simulink library "commsrccod"  (Simulink 5.0)
libraries: commsrccod x2
settings Model: Creator=mikem  LastModifiedBy=mmclerno

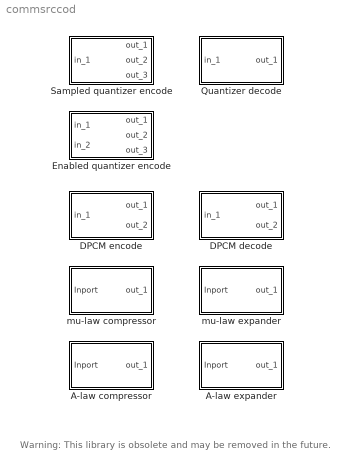
== system commsrccod ==
  note: Warning:  This library is obsolete and may be
      | removed in the future.
  A-law compressor : Subsystem  mask(A-law compressor){A=87.6, V=1}
      mask prompts: A "A value:"; V "Peak signal magnitude:"
      mask help: Compress the input signal using A-law compressor. The A-law compressor uses logarithm computation.
      mask init:
      | lnA1=log(A)+1;AdlnA1=A/lnA1;VdlnA1=V/lnA1;VdA=V/A;AdV=A/V;
      mask Help: This block processes a vector signal. The output has the same length as the input signal. The prevailing value for A is A=87.6.
      mask Display: disp('A-law\ncompressor')
  A-law expander : Subsystem  mask(A-law expander){A=87.6, V=1}
      mask prompts: A "A value:"; V "Signal peak magnitude:"
      mask help: Inverse computation of A-law compressor.
      mask init:
      | lnA1=log(A)+1;VdlnA1=V/lnA1;lnA1dA=lnA1/A;lnA1dV=lnA1/V;VdA=V/A;
      mask Help: This block reverses the computation with A-law compressor. The prevailing value for A is A=87.6.
      mask Display: disp('A-law\nexpander')
  DPCM decode : Subsystem  mask(DPCM decode){num=[0 .9963], den=1, codebook=[-.0848 -.029 .0298 .0853], sample_time=.1}
      mask prompts: num "Predictor transfer function numerator:"; den "Predictor transfer function denominator:"; codebook "Quantization codebook:"; sample_time "Sample time (sec):"
      mask help: Input the DPCM coded index. Output DPCM decodes to the 1st outport and quantization decode to the 2nd outport.
      mask Help: This block recovers the source code using the DPCM decode method. The parameters in this block should match the parameters in the DPCM encoder.
      mask Display: disp('DPCM\ndecode')
  DPCM encode : Subsystem  mask(DPCM encode){num=[0 .9963], den=1, partition=[-.0569 .0004 .0576], codebook=[-.0848 -.029 .0298 .0853], sample_time=.1}
      mask prompts: num "Predictor numerator:"; den "Predictor denominator:"; partition "Quantization partition:"; codebook "Quantization codebook:"; sample_time "Sample time (sec):"
      mask help: Output the DPCM encoded index to the 1st outport and the quantization recovered value to the 2nd outport.
      mask Help: The 1st outport outputs the index of the predictive error. The 2nd outport outputs the predictive error. Use the DPCMOPT function for the FIR filter training. A delta modulation is a special case with the numerator as [0,x], the denominator as 1 for the\npredictor.
      mask Display: disp('DPCM\nencode')
  Enabled quantizer encode : Subsystem  mask(Scalar quantization encode){partition=[-.75 -.25 .25 .75], codebook=[-.825 -.5 0 .5 .825], n=2}
      mask prompts: partition "Quantization partition:"; codebook "Quantization codebook:"; n "Input signal vector length:"
      mask help: Triggered by 2nd input signal, this block quantize an analog signal to (1)digital signal, (2)quantization value, (3)distortion.
      mask init:
      | [x,y]=trigicon(0,25,get_param(gcb,'orientation'),1);
      mask Help: This block quantizes the first inport signal into quantization index (1st outport), quantized value (2nd outport), and distortion (3rd outport). This block uses scalar quantization method. The input signal to the 1st inport can be a vector. The operation of this block is enabled by the non-zero signal from the second inport. When the block is not enabled, the block keeps the last output value.
      mask Display: plot(0,0,100,100,x,y);disp('Quantizer')
  Quantizer decode : Subsystem  mask(Scalar quantization decode){codebook=[-.825 -.5 0, .5 .825]}
      mask prompts: codebook "Quantization codebook:"
      mask help: Output the value in the given codebook based on the input index value.
      mask Help: This block takes the quantized index as input and outputs the quantization value. The output vector size is the same as the input vector size. Inputs 0, 1, ..., N-1 lead to CK(1), CK(2), .. CK(N) output.
      mask Display: disp('Quantizer\ndecode')
  Sampled quantizer encode : Subsystem  mask(Scalar quantization encode){partition=[-.75 -.25 .25 .75], codebook=[-.825 -.5 0 .5 .825], n=2, sample_time=.1}
      mask prompts: partition "Quantization partition:"; codebook "Quantization codebook:"; n "Input signal vector length:"; sample_time "Sample time (sec):"
      mask help: Quantize an analog signal to (1)digital signal, (2)quantization value, and (3)distortion at every sample time point.
      mask Help: This block converts the input analog signal to digital signal (1st outport) with the quantized value (2nd outport), and distortion (3rd outport) at every sample point. The input signa can be a vector. When the sample time is a two-elements vector, the second element is the offset value. The length of the partition is one less than the length of codebook. Use LLOYDS to optimize the partition and codebook.
      mask Display: disp('Scalar\nquantizer')
  mu-law compressor : Subsystem  mask(mu-law compressor){mu=255, V=1}
      mask prompts: mu "mu value:"; V "Peak signal magnitude:"
      mask help: Compress the input signal using mu-law compressor. The mu-law compressor uses logarithm computation.
      mask init:
      | mudV=mu/V;Vln1mu=V/log(1+mu);
      mask Help: This block processes a vector signal. The output has the same length as the input signal. The prevailing value is mu=255.
      mask Display: disp('mu-law\ncompressor')
  mu-law expander : Subsystem  mask(mu-law expander){mu=255, V=1}
      mask prompts: mu "mu value:"; V "Signal peak magnitude:"
      mask help: Inverse computation of mu-law compressor.
      mask init:
      | Vmu=V/mu;ln1mdV=log(1+mu)/V;
      mask Help: This block reverses the computation with mu-law compressor. The prevailing value for mu is mu=255.
      mask Display: disp('mu-law\nexpander')

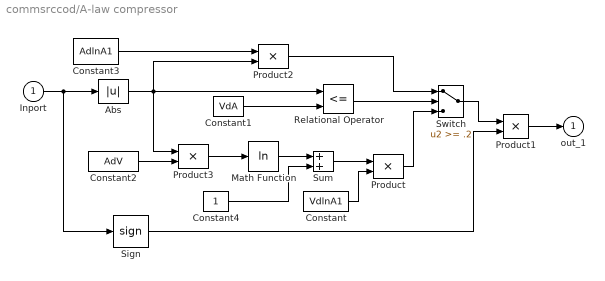
== system commsrccod/A-law compressor ==
  Inport : Inport
  Abs : Abs  SaturateOnIntegerOverflow=on
  Constant : Constant  Value=VdlnA1
  Constant1 : Constant  Value=VdA
  Constant2 : Constant  Value=AdV
  Constant3 : Constant  Value=AdlnA1
  Constant4 : Constant
  Math Function : Math  Operator=log
  Product{,1..3} (4 alike) : Product  SaturateOnIntegerOverflow=on  InputSameDT=on
  Relational Operator : RelationalOperator  Operator=<=  InputSameDT=on
  Sign : Signum
  Sum : Sum  SaturateOnIntegerOverflow=on  InputSameDT=on
  Switch : Switch  Threshold=.2  SaturateOnIntegerOverflow=on  InputSameDT=on
  out_1 : Outport  InitialOutput=0
  wires:
  Product1/1 -> out_1/1
  Inport/1 -> Sign/1, Abs/1
  Sign/1 -> Product1/2
  Switch/1 -> Product1/1
  Constant1/1 -> Relational Operator/2
  Relational Operator/1 -> Switch/2
  Product2/1 -> Switch/1
  Constant3/1 -> Product2/1
  Constant2/1 -> Product3/2
  Abs/1 -> Product3/1, Product2/2, Relational Operator/1
  Product3/1 -> Math Function/1
  Math Function/1 -> Sum/1
  Constant4/1 -> Sum/2
  Constant/1 -> Product/2
  Sum/1 -> Product/1
  Product/1 -> Switch/3

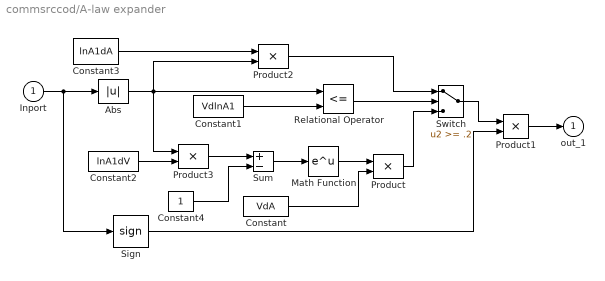
== system commsrccod/A-law expander ==
  Inport : Inport
  Abs : Abs  SaturateOnIntegerOverflow=on
  Constant : Constant  Value=VdA
  Constant1 : Constant  Value=VdlnA1
  Constant2 : Constant  Value=lnA1dV
  Constant3 : Constant  Value=lnA1dA
  Constant4 : Constant
  Math Function : Math
  Product{,1..3} (4 alike) : Product  SaturateOnIntegerOverflow=on  InputSameDT=on
  Relational Operator : RelationalOperator  Operator=<=  InputSameDT=on
  Sign : Signum
  Sum : Sum  Inputs=+-  SaturateOnIntegerOverflow=on  InputSameDT=on
  Switch : Switch  Threshold=.2  SaturateOnIntegerOverflow=on  InputSameDT=on
  out_1 : Outport  InitialOutput=0
  wires:
  Product/1 -> Switch/3
  Constant/1 -> Product/2
  Constant4/1 -> Sum/2
  Constant2/1 -> Product3/2
  Constant3/1 -> Product2/1
  Product2/1 -> Switch/1
  Abs/1 -> Product3/1, Product2/2, Relational Operator/1
  Relational Operator/1 -> Switch/2
  Constant1/1 -> Relational Operator/2
  Switch/1 -> Product1/1
  Sign/1 -> Product1/2
  Inport/1 -> Sign/1, Abs/1
  Product1/1 -> out_1/1
  Product3/1 -> Sum/1
  Sum/1 -> Math Function/1
  Math Function/1 -> Product/1

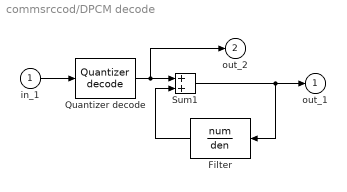
== system commsrccod/DPCM decode ==
  in_1 : Inport
  Filter : DiscreteFilter  Orientation=left  Numerator=num  Denominator=den  SampleTime=sample_time
  Quantizer decode : commsrccod/Quantizer decode  codebook=codebook
  Sum1 : Sum  SaturateOnIntegerOverflow=on  InputSameDT=on
  out_1 : Outport  InitialOutput=0
  out_2 : Outport  Port=2  InitialOutput=0
  wires:
  Quantizer decode/1 -> out_2/1, Sum1/1
  Sum1/1 -> Filter/1, out_1/1
  Filter/1 -> Sum1/2
  in_1/1 -> Quantizer decode/1

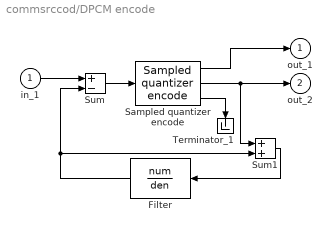
== system commsrccod/DPCM encode ==
  in_1 : Inport
  Filter : DiscreteFilter  Orientation=left  Numerator=num  Denominator=den  SampleTime=sample_time
  Sampled quantizer encode : commsrccod/Sampled quantizer encode  partition=partition  codebook=codebook  n=1  sample_time=sample_time
  Sum : Sum  Inputs=+-  SaturateOnIntegerOverflow=on  InputSameDT=on
  Sum1 : Sum  SaturateOnIntegerOverflow=on  InputSameDT=on
  Terminator_1 : Terminator
      settings: Orientation=down
  out_1 : Outport  InitialOutput=0
  out_2 : Outport  Port=2  InitialOutput=0
  wires:
  Sampled quantizer encode/3 -> Terminator_1/1
  Sampled quantizer encode/2 -> out_2/1, Sum1/1
  Sampled quantizer encode/1 -> out_1/1
  Sum/1 -> Sampled quantizer encode/1
  in_1/1 -> Sum/1
  Filter/1 -> Sum1/2, Sum/2
  Sum1/1 -> Filter/1

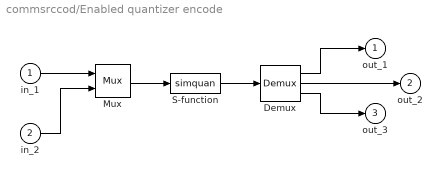
== system commsrccod/Enabled quantizer encode ==
  in_1 : Inport
  in_2 : Inport  Port=2
  Demux : Demux  Outputs=[n n n]
  Mux : Mux  Inputs=[n 1]
  S-function : S-Function  FunctionName=simquan  Parameters=n, partition, codebook
  out_1 : Outport  InitialOutput=0
  out_2 : Outport  Port=2  InitialOutput=0
  out_3 : Outport  Port=3  InitialOutput=0
  wires:
  Demux/3 -> out_3/1
  Demux/2 -> out_2/1
  Demux/1 -> out_1/1
  S-function/1 -> Demux/1
  Mux/1 -> S-function/1
  in_2/1 -> Mux/2
  in_1/1 -> Mux/1

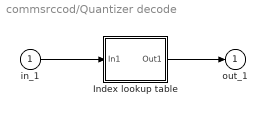
== system commsrccod/Quantizer decode ==
  in_1 : Inport
  Index lookup table : Subsystem  mask(No-intepret Lookup table){@1=codebook}
      mask prompts: @1 "Codebook:"
      mask help: Output one of the values in the look-up table.
      mask init:
      | codebook=@1;
      mask Help: When codebook is a matrix, the block input can only be a scalar. The block output the row with the column index provided in the input. When codebook is a vector, the block output the same length as the input vector. The output is one of the values in codebook with the index provided by the input.
      mask Display: disp('Index\nLookup tb')
  out_1 : Outport  InitialOutput=0
  wires:
  Index lookup table/1(Out1) -> out_1/1
  in_1/1 -> Index lookup table/1(In1)

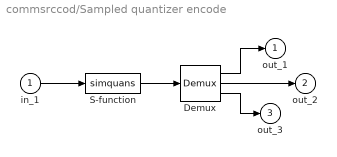
== system commsrccod/Sampled quantizer encode ==
  in_1 : Inport
  Demux : Demux  Outputs=[n n n]
  S-function : S-Function  FunctionName=simquans  Parameters=n, partition, codebook,sample_time
  out_1 : Outport  InitialOutput=0
  out_2 : Outport  Port=2  InitialOutput=0
  out_3 : Outport  Port=3  InitialOutput=0
  wires:
  in_1/1 -> S-function/1
  S-function/1 -> Demux/1
  Demux/1 -> out_1/1
  Demux/2 -> out_2/1
  Demux/3 -> out_3/1

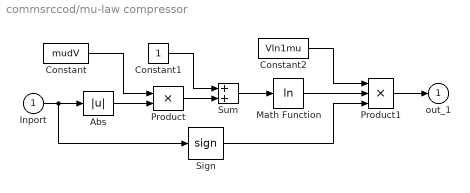
== system commsrccod/mu-law compressor ==
  Inport : Inport
  Abs : Abs  SaturateOnIntegerOverflow=on
  Constant : Constant  Value=mudV
  Constant1 : Constant
  Constant2 : Constant  Value=Vln1mu
  Math Function : Math  Operator=log
  Product : Product  SaturateOnIntegerOverflow=on  InputSameDT=on
  Product1 : Product  Inputs=3  SaturateOnIntegerOverflow=on  InputSameDT=on
  Sign : Signum
  Sum : Sum  SaturateOnIntegerOverflow=on  InputSameDT=on
  out_1 : Outport  InitialOutput=0
  wires:
  Product1/1 -> out_1/1
  Constant2/1 -> Product1/1
  Sign/1 -> Product1/3
  Math Function/1 -> Product1/2
  Inport/1 -> Sign/1, Abs/1
  Sum/1 -> Math Function/1
  Constant1/1 -> Sum/1
  Product/1 -> Sum/2
  Constant/1 -> Product/1
  Abs/1 -> Product/2

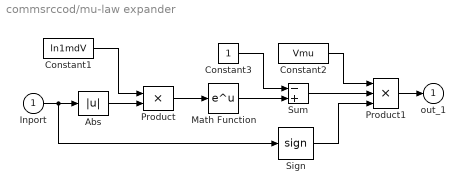
== system commsrccod/mu-law expander ==
  Inport : Inport
  Abs : Abs  SaturateOnIntegerOverflow=on
  Constant1 : Constant  Value=ln1mdV
  Constant2 : Constant  Value=Vmu
  Constant3 : Constant
  Math Function : Math
  Product : Product  SaturateOnIntegerOverflow=on  InputSameDT=on
  Product1 : Product  Inputs=3  SaturateOnIntegerOverflow=on  InputSameDT=on
  Sign : Signum
  Sum : Sum  Inputs=-+  SaturateOnIntegerOverflow=on  InputSameDT=on
  out_1 : Outport  InitialOutput=0
  wires:
  Constant3/1 -> Sum/1
  Sum/1 -> Product1/2
  Math Function/1 -> Sum/2
  Product1/1 -> out_1/1
  Sign/1 -> Product1/3
  Inport/1 -> Sign/1, Abs/1
  Constant2/1 -> Product1/1
  Product/1 -> Math Function/1
  Abs/1 -> Product/2
  Constant1/1 -> Product/1

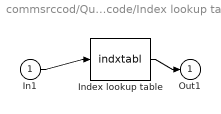
== system commsrccod/Quantizer decode/Index lookup table ==
  In1 : Inport
  Index lookup table : S-Function  FunctionName=indxtabl  Parameters=codebook
  Out1 : Outport  InitialOutput=0
  wires:
  In1/1 -> Index lookup table/1
  Index lookup table/1 -> Out1/1
